simulink library "lib_darwinop_2011a"  (Simulink 7.7)
settings: Solver=ode45  StartTime=0.0  StopTime=10.0  RelTol=1e-3
undefined symbols (not defined in the file or in its folder): darwinop_communication_setup, usb2dynamixel_communication_setup
libraries: simulink x1
settings Model: Creator=florent  LastModifiedBy=eleve

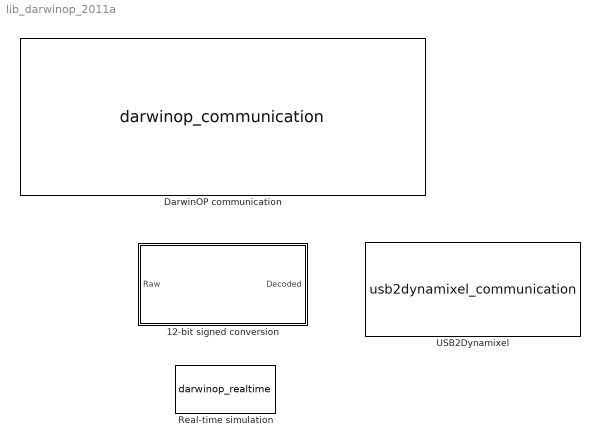
== system lib_darwinop_2011a ==
  12-bit signed conversion : Subsystem  TreatAsAtomicUnit=on
      mask Type: Datatype conversion
      mask Description: Convert Dynamixel raw speed and load values to signed numbers.
      mask Display:
      | image(imread('darwin-conversion.jpg'))
      | 
      | port_label('output',1,'Decoded')
      | port_label('input',1,'Raw')
  DarwinOP communication : M-S-Function  StartFcn=darwinop_communication_setup('StartFcn');  StopFcn=darwinop_communication_setup('StopFcn');  FunctionName=darwinop_communication  Parameters=IP,Port,Protocol,SampleTime,Frame,ReadIndex,WriteIndex  mask{IP=192.168.123.1, Port=1234, Protocol=tcp, SampleTime=0.5, Frame=[ 2 1 36 6 3 1 30 2 0 0 2 200 44 6], ReadIndex=[ 1 2;3 2;5 2;7 2;9 2;11 2], WriteIndex=[ 9 2]}
      settings: DeleteFcn=darwinop_communication_setup('DeleteFcn');  ModelCloseFcn=darwinop_communication_setup('ModelCloseFcn');  NameChangeFcn=darwinop_communication_setup('NameChangeFcn');  OpenFcn=darwinop_communication_setup('OpenFcn');
      mask StyleString: edit,edit,popup(tcp|udp),edit,edit,edit,edit
      mask Display:
      | image(imread('darwin-blk.jpg'))
      | 
      | port_label('output',1,'Right Shoulder Pitch(1)/Position')
      | port_label('output',2,'Right Shoulder Pitch(1)/Speed')
      | port_label('output',3,'Right Shoulder Pitch(1)/Load')
      | port_label('output',4,'Sub controller(200)/ACC X')
      | port_label('output',5,'Sub controller(200)/ACC Y')
      | port_label('output',6,'Sub controller(200)/ACC Z')
      | 
      | port_label('input',1,'Right Shoulder Pitch(1)/Goal Position')
  Real-time simulation : M-S-Function  FunctionName=darwinop_realtime  Parameters=TimeScalingFactor  mask(Real-time simulation parameters ){TimeScalingFactor=1}
      mask prompts: TimeScalingFactor "Scaling Factor:"
      mask help: At each simulation step, this block ensures the simulation time is synchronized with the clock, resulting in a soft real-time simulation (with skews).
      mask Display: fprintf('Scaling factor = %d', TimeScalingFactor)
  USB2Dynamixel : M-S-Function  StartFcn=usb2dynamixel_communication_setup('StartFcn');  StopFcn=usb2dynamixel_communication_setup('StopFcn');  FunctionName=usb2dynamixel_communication  Parameters=COMPort,BaudRate,SampleTime,Frame,ReadIndex,WriteIndex,DisableStatusReturn  mask{COMPort='COM11', BaudRate=1000000, SampleTime=0.05, Frame=[ 2 10 36 6 3 10 30 2 0 0], ReadIndex=[ 1 2;3 2;5 2], WriteIndex=[ 9 2], DisableStatusReturn=0}
      settings: DeleteFcn=usb2dynamixel_communication_setup('DeleteFcn');  ModelCloseFcn=usb2dynamixel_communication_setup('ModelCloseFcn');  NameChangeFcn=usb2dynamixel_communication_setup('NameChangeFcn');  OpenFcn=usb2dynamixel_communication_setup('OpenFcn');
      mask Display:
      | image(imread('usb2dynamixel.jpg'))
      | 
      | port_label('output',1,'RX24F(10)/Position')
      | port_label('output',2,'RX24F(10)/Speed')
      | port_label('output',3,'RX24F(10)/Load')
      | 
      | port_label('input',1,'RX24F(10)/Goal Position')

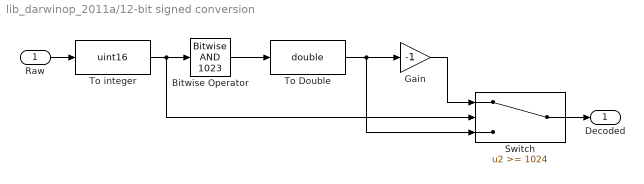
== system lib_darwinop_2011a/12-bit signed conversion ==
  Raw : Inport
  Bitwise Operator : simulink/Logic and Bit Operations/Bitwise Operator  logicop=AND  UseBitMask=on  BitMask=1023  BitMaskRealWorld=Stored Integer
  Gain : Gain  Gain=-1
  Switch : Switch  Threshold=1024
  To Double : DataTypeConversion  OutDataTypeStr=double
  To integer : DataTypeConversion  OutDataTypeStr=uint16
  Decoded : Outport
  wires:
  Raw/1 -> To integer/1
  To integer/1 -> Switch/2, Bitwise Operator/1
  Bitwise Operator/1 -> To Double/1
  To Double/1 -> Switch/3, Gain/1
  Switch/1 -> Decoded/1
  Gain/1 -> Switch/1
